simulink model "FDIBenchMark_66"  (Simulink 7.0)
settings: Solver=ode45  StartTime=0.0  StopTime=4400  FixedStep=Ts  RelTol=1e-12
InitFcn:
  | FDIBenchMarkData
values from neighbouring files (symbols this model uses):
  a = 2.2    [FDIBenchMarkData.m]
  Addt = [-(B_dt+B_r)/J_r B_dt/N_g/J_r -K_dt/J_r; eta_dt*B_dt/N_g/J_g -(eta_dt*B_dt/N_g^2+B_g)/J_g eta_dt*K_dt/N_g/J_g; 1 -1/N_g 0]    [FDIBenchMarkData.m]
  Addt2 = [-(B_dt+B_r)/J_r B_dt/N_g/J_r -K_dt/J_r; eta_dt2*B_dt/N_g/J_g -(eta_dt2*B_dt/N_g^2+B_g)/J_g eta_dt2*K_dt/N_g/J_g; 1 -1/N_g 0]    [FDIBenchMarkData.m]
  alpha = 0.1    [FDIBenchMarkData.m]
  alpha_gc = 50    [FDIBenchMarkData.m]
  Bddt = [1/J_r 0; 0 -1/J_g;0 0]    [FDIBenchMarkData.m]
  Bddt2 = [1/J_r 0; 0 -1/J_g;0 0]    [FDIBenchMarkData.m]
  Cddt = [1 0 0;0 1 0]    [FDIBenchMarkData.m]
  Constant_Beta_1_m1 = 5    [FDIBenchMarkData.m]
  Constant_Beta_3_m1 = 10    [FDIBenchMarkData.m]
  Constant_Omega_r_m1 = 1.4    [FDIBenchMarkData.m]
  Constant_tau_gc = 100    [FDIBenchMarkData.m]
  eta_gc = 0.98    [FDIBenchMarkData.m]
  Gain_Beta_2_m2 = 1.2    [FDIBenchMarkData.m]
  Gain_Omega_r_m2 = 1.1    [FDIBenchMarkData.m]
  H = 87    [FDIBenchMarkData.m]
  k = 4.7    [FDIBenchMarkData.m]
  K_i = 1    [FDIBenchMarkData.m]
  K_opt = .5* rho* pi*R^2*eta_dt*R^3*0.4554/(N_g*8)^3    (= 1.21708013189)    [FDIBenchMarkData.m]
  K_p = 4    [FDIBenchMarkData.m]
  L = acker(A', C', vpe)'    [FDIBenchMarkData.m]
  m = 1+alpha*(alpha-1)*R^2/(8*H^2)    (= 0.995085835315)    [FDIBenchMarkData.m]
  m_Beta = 0    [FDIBenchMarkData.m]
  m_omega_g = 0    [FDIBenchMarkData.m]
  m_omega_r = 0    [FDIBenchMarkData.m]
  m_P_g = 0    [FDIBenchMarkData.m]
  m_tau_g = 0    [FDIBenchMarkData.m]
  m_vw = 1.5    [FDIBenchMarkData.m]
  Omega_delta = 15    [FDIBenchMarkData.m]
  omega_n = 11.11    [FDIBenchMarkData.m]
  Omega_nom = 162    [FDIBenchMarkData.m]
  P_r = 4.8e6    (= 4800000)    [FDIBenchMarkData.m]
  R = 57.5    [FDIBenchMarkData.m]
  r = D_rotor/2    (= 57.5)    [FDIBenchMarkData.m]
  r0 = 1.5    [FDIBenchMarkData.m]
  rho = 1.225    [FDIBenchMarkData.m]
  seed = ceil(seed)    [FDIBenchMarkData.m]
  sigma_Beta = 0.2    [FDIBenchMarkData.m]
  sigma_omega_g = 0.05    [FDIBenchMarkData.m]
  sigma_omega_r = 0.004*2*pi    (= 0.0251327412287)    [FDIBenchMarkData.m]
  sigma_P_g = 1e3    (= 1000)    [FDIBenchMarkData.m]
  sigma_tau_g = 90    [FDIBenchMarkData.m]
  sigma_vm = 0.5    [FDIBenchMarkData.m]
  T_sample = 0.05    [FDIBenchMarkData.m]
  Ts = 1/100    (= 0.01)    [FDIBenchMarkData.m]
  turb_int = Turbulence_intensity    (= 12)    [FDIBenchMarkData.m]
  turbulence_seeds = [seed1 seed2]    [FDIBenchMarkData.m]
  xi = 0.6    [FDIBenchMarkData.m]
undefined symbols (not defined in the file or in its folder): Apb, Apb1, Apb2, Bpb, Bpb1, Bpb2, Cpb, Cpb1, Cpb2, Cq, DiscIntNeverNeededParam, u0
(part 2 of 2)

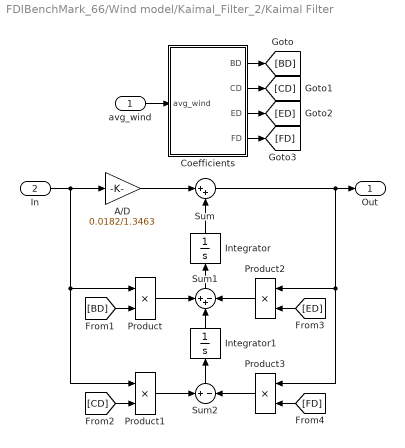
== system FDIBenchMark_66/Wind model/Kaimal_Filter_2/Kaimal Filter ==
  avg_wind : Inport  OutDataType=sfix(16)  OutScaling=2^0
  In : Inport  Port=2  OutDataType=sfix(16)  OutScaling=2^0
  A/D : Gain  Gain=0.0182/1.3463  ParameterDataType=sfix(16)  ParameterScaling=2^0  OutDataType=sfix(16)  OutScaling=2^0  SaturateOnIntegerOverflow=on
  Coefficients : Subsystem
  Integrator : Integrator  Orientation=up
  Integrator1 : Integrator  Orientation=up
  Product : Product  OutDataType=sfix(16)  OutScaling=2^0  SaturateOnIntegerOverflow=on
  Product1 : Product  OutDataType=sfix(16)  OutScaling=2^0  SaturateOnIntegerOverflow=on
  Product2 : Product  Orientation=left  OutDataType=sfix(16)  OutScaling=2^0  SaturateOnIntegerOverflow=on
  Product3 : Product  Orientation=left  OutDataType=sfix(16)  OutScaling=2^0  SaturateOnIntegerOverflow=on
  Sum : Sum  Inputs=|++  OutDataType=sfix(16)  OutScaling=2^0  SaturateOnIntegerOverflow=on
  Sum1 : Sum  Orientation=up  Inputs=++-  OutDataType=sfix(16)  OutScaling=2^0  SaturateOnIntegerOverflow=on
  Sum2 : Sum  Orientation=up  Inputs=+|-  OutDataType=sfix(16)  OutScaling=2^0  SaturateOnIntegerOverflow=on
  Out : Outport  OutDataType=sfix(16)  OutScaling=2^0
  wires:
  A/D/1 -> Sum/1
  Integrator/1 -> Sum/2
  Sum1/1 -> Integrator/1
  Product/1 -> Sum1/1
  Integrator1/1 -> Sum1/2
  Product2/1 -> Sum1/3
  Sum2/1 -> Integrator1/1
  Product3/1 -> Sum2/2
  Product1/1 -> Sum2/1
  Sum/1 -> Product2/1, Product3/1, Out/1
  In/1 -> A/D/1, Product/1, Product1/1
  [BD] -> Product/2
  [CD] -> Product1/2
  [ED] -> Product2/2
  [FD] -> Product3/2
  Coefficients/1(BD) -> [BD]
  Coefficients/2(CD) -> [CD]
  Coefficients/3(ED) -> [ED]
  Coefficients/4(FD) -> [FD]
  avg_wind/1 -> Coefficients/1(avg_wind)

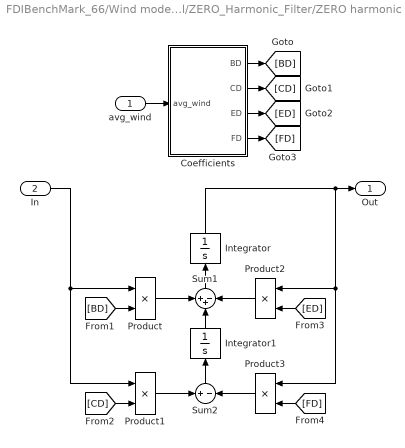
== system FDIBenchMark_66/Wind model/ZERO_Harmonic_Filter/ZERO harmonic Filter ==
  avg_wind : Inport  OutDataType=sfix(16)  OutScaling=2^0
  In : Inport  Port=2  OutDataType=sfix(16)  OutScaling=2^0
  Coefficients : Subsystem
  Integrator : Integrator  Orientation=up
  Integrator1 : Integrator  Orientation=up
  Product : Product  OutDataType=sfix(16)  OutScaling=2^0  SaturateOnIntegerOverflow=on
  Product1 : Product  OutDataType=sfix(16)  OutScaling=2^0  SaturateOnIntegerOverflow=on
  Product2 : Product  Orientation=left  OutDataType=sfix(16)  OutScaling=2^0  SaturateOnIntegerOverflow=on
  Product3 : Product  Orientation=left  OutDataType=sfix(16)  OutScaling=2^0  SaturateOnIntegerOverflow=on
  Sum1 : Sum  Orientation=up  Inputs=++-  OutDataType=sfix(16)  OutScaling=2^0  SaturateOnIntegerOverflow=on
  Sum2 : Sum  Orientation=up  Inputs=+|-  OutDataType=sfix(16)  OutScaling=2^0  SaturateOnIntegerOverflow=on
  Out : Outport  OutDataType=sfix(16)  OutScaling=2^0
  wires:
  Integrator/1 -> Product2/1, Product3/1, Out/1
  Sum1/1 -> Integrator/1
  Product/1 -> Sum1/1
  Integrator1/1 -> Sum1/2
  Product2/1 -> Sum1/3
  Sum2/1 -> Integrator1/1
  Product3/1 -> Sum2/2
  Product1/1 -> Sum2/1
  In/1 -> Product/1, Product1/1
  [BD] -> Product/2
  [CD] -> Product1/2
  [ED] -> Product2/2
  [FD] -> Product3/2
  Coefficients/1(BD) -> [BD]
  Coefficients/2(CD) -> [CD]
  Coefficients/3(ED) -> [ED]
  Coefficients/4(FD) -> [FD]
  avg_wind/1 -> Coefficients/1(avg_wind)

== system FDIBenchMark_66/Wind model/3rd_Harmonic_Filter1/3rd harmonic Filter/Coefficients ==
  avg_wind : Inport  OutDataType=sfix(16)  OutScaling=2^0
  BD coeff : Fcn  Expr=0.2766/0.3691/(r/u(1))
  CD coeff : Fcn  Expr=0.0307/0.3691/(r/u(1))^2
  ED coeff : Fcn  Expr=1.7722/0.3691/(r/u(1))
  FD coeff : Fcn  Expr=1/0.3691/(r/u(1))^2
  BD : Outport  OutDataType=sfix(16)  OutScaling=2^0
  CD : Outport  Port=2  OutDataType=sfix(16)  OutScaling=2^0
  ED : Outport  Port=3  OutDataType=sfix(16)  OutScaling=2^0
  FD : Outport  Port=4  OutDataType=sfix(16)  OutScaling=2^0
  wires:
  FD coeff/1 -> FD/1
  ED coeff/1 -> ED/1
  CD coeff/1 -> CD/1
  BD coeff/1 -> BD/1
  avg_wind/1 -> FD coeff/1, ED coeff/1, CD coeff/1, BD coeff/1

== system FDIBenchMark_66/Wind model/Kaimal_Filter_1/Kaimal Filter/Coefficients ==
  avg_wind : Inport  OutDataType=sfix(16)  OutScaling=2^0
  BD coeff : Fcn  Expr=1.3653/1.3463/(L/2/pi/u(1))
  CD coeff : Fcn  Expr=0.9846/1.3463/(L/2/pi/u(1))^2
  ED coeff : Fcn  Expr=3.7593/1.3463/(L/2/pi/u(1))
  FD coeff : Fcn  Expr=1/1.3463/(L/2/pi/u(1))^2
  BD : Outport  OutDataType=sfix(16)  OutScaling=2^0
  CD : Outport  Port=2  OutDataType=sfix(16)  OutScaling=2^0
  ED : Outport  Port=3  OutDataType=sfix(16)  OutScaling=2^0
  FD : Outport  Port=4  OutDataType=sfix(16)  OutScaling=2^0
  wires:
  FD coeff/1 -> FD/1
  ED coeff/1 -> ED/1
  CD coeff/1 -> CD/1
  BD coeff/1 -> BD/1
  avg_wind/1 -> FD coeff/1, ED coeff/1, CD coeff/1, BD coeff/1

== system FDIBenchMark_66/Wind model/Kaimal_Filter_2/Kaimal Filter/Coefficients ==
  avg_wind : Inport  OutDataType=sfix(16)  OutScaling=2^0
  BD coeff : Fcn  Expr=1.3653/1.3463/(L/2/pi/u(1))
  CD coeff : Fcn  Expr=0.9846/1.3463/(L/2/pi/u(1))^2
  ED coeff : Fcn  Expr=3.7593/1.3463/(L/2/pi/u(1))
  FD coeff : Fcn  Expr=1/1.3463/(L/2/pi/u(1))^2
  BD : Outport  OutDataType=sfix(16)  OutScaling=2^0
  CD : Outport  Port=2  OutDataType=sfix(16)  OutScaling=2^0
  ED : Outport  Port=3  OutDataType=sfix(16)  OutScaling=2^0
  FD : Outport  Port=4  OutDataType=sfix(16)  OutScaling=2^0
  wires:
  avg_wind/1 -> BD coeff/1, CD coeff/1, ED coeff/1, FD coeff/1
  BD coeff/1 -> BD/1
  CD coeff/1 -> CD/1
  ED coeff/1 -> ED/1
  FD coeff/1 -> FD/1

== system FDIBenchMark_66/Wind model/ZERO_Harmonic_Filter/ZERO harmonic Filter/Coefficients ==
  avg_wind : Inport  OutDataType=sfix(16)  OutScaling=2^0
  BD coeff : Fcn  Expr=4.7869/7.6823/(r/u(1))
  CD coeff : Fcn  Expr=0.9904/7.6823/(r/u(1))^2
  ED coeff : Fcn  Expr=7.3518/7.6823/(r/u(1))
  FD coeff : Fcn  Expr=1/7.6823/(r/u(1))^2
  BD : Outport  OutDataType=sfix(16)  OutScaling=2^0
  CD : Outport  Port=2  OutDataType=sfix(16)  OutScaling=2^0
  ED : Outport  Port=3  OutDataType=sfix(16)  OutScaling=2^0
  FD : Outport  Port=4  OutDataType=sfix(16)  OutScaling=2^0
  wires:
  avg_wind/1 -> BD coeff/1, CD coeff/1, ED coeff/1, FD coeff/1
  BD coeff/1 -> BD/1
  CD coeff/1 -> CD/1
  ED coeff/1 -> ED/1
  FD coeff/1 -> FD/1

== matlab function Controller/Embedded MATLAB Function ==
  data: P_g input inherited; ControlZone output inherited; P_r input inherited; Omega_g input inherited; LastControlZone input inherited; Omega_nom input inherited; Omega_delta input inherited
function ControlZone = ZoneControl(P_g, P_r, Omega_g, LastControlZone,Omega_nom,Omega_delta)
 
if LastControlZone==0,
    if (P_g>=P_r) || (Omega_g>=Omega_nom)
        ControlZone=1;
    else
        ControlZone=0;
    end
else
    if (Omega_g<(Omega_nom-Omega_delta))
        ControlZone=0;
    else
        ControlZone=1;
    end
end
